simulink subsystem "MCU"  (R2023a)
settings: Solver=VariableStepAuto  StartTime=0.0  StopTime=10.0  RelTol=1e-3
settings Model: Creator=hidra  LastModifiedBy=hidra

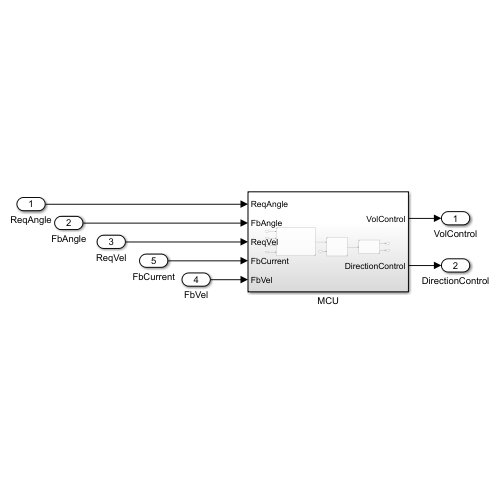
[thumbnail: Simulink's stored preview of the top-level diagram]
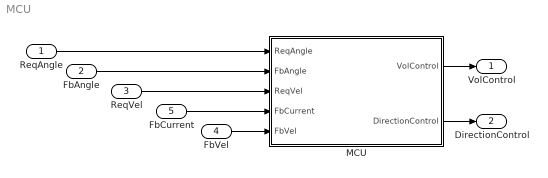
== system MCU ==
  ReqAngle : Inport
  FbAngle : Inport  Port=2
  ReqVel : Inport  Port=3
  FbVel : Inport  Port=4
  FbCurrent : Inport  Port=5
  MCU : Subsystem
  VolControl : Outport
  DirectionControl : Outport  Port=2
  wires:
  ReqAngle/1 -> MCU/1(ReqAngle)
  FbAngle/1 -> MCU/2(FbAngle)
  ReqVel/1 -> MCU/3(ReqVel)
  FbCurrent/1 -> MCU/4(FbCurrent)
  FbVel/1 -> MCU/5(FbVel)
  MCU/1(VolControl) -> VolControl/1
  MCU/2(DirectionControl) -> DirectionControl/1

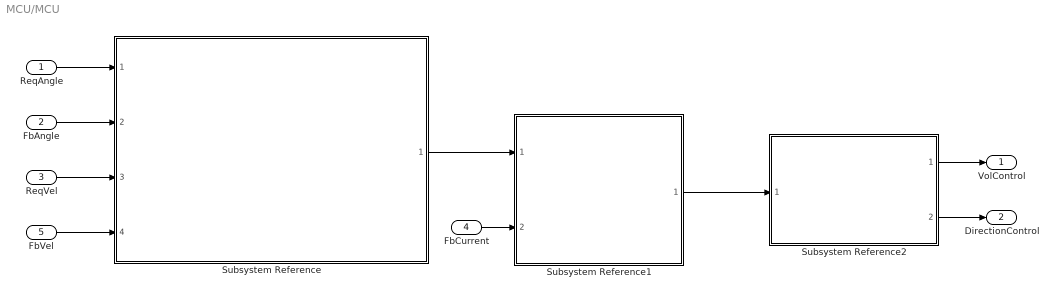
== system MCU/MCU ==
  ReqAngle : Inport
  FbAngle : Inport  Port=2
  ReqVel : Inport  Port=3
  FbCurrent : Inport  Port=4
  FbVel : Inport  Port=5
  Subsystem Reference : Subsystem  ReferencedSubsystem=HighLevelController
  Subsystem Reference1 : Subsystem  ReferencedSubsystem=LowLevelController1
  Subsystem Reference2 : Subsystem  ReferencedSubsystem=CONTROLADAPTER_
  VolControl : Outport
  DirectionControl : Outport  Port=2
  wires:
  FbAngle/1 -> Subsystem Reference/2
  Subsystem Reference1/1 -> Subsystem Reference2/1
  FbVel/1 -> Subsystem Reference/4
  Subsystem Reference/1 -> Subsystem Reference1/1
  ReqVel/1 -> Subsystem Reference/3
  ReqAngle/1 -> Subsystem Reference/1
  FbCurrent/1 -> Subsystem Reference1/2
  Subsystem Reference2/2 -> DirectionControl/1
  Subsystem Reference2/1 -> VolControl/1
